simulink model "PMSM_SVC_HF"  (R2023a)
settings: Solver=ode1  StartTime=0.0  StopTime=7  FixedStep=Tsim  RelTol=1e-3  EnableMultiTasking=on
InitFcn:
  | %% Parameters of the motor
  | Pw_n = 1;                                                                   % The nominal power of the SM (kW)
  | Ull_n = 380;                                                                % The nominal line-line voltage (Vrms)
  | I_n = 2;                                                                    % The nominal current (A)
  | f_n = 50;                                                                   % The nominal frequency (Hz)
  | N_n = 1500;                                                                 % The nominal rotation speed of motor (rad.min^-1)
  | p = 2;                                                                      % Pole pairs
  | T_n = 5;                                                                    % The nominal torque of motor (N.m)
  | 
  | Rs = 0.91;                                                                  % The stator resistance (ohm)
  | Ld = 3.96e-3;                                                               % The d-axis inductance (H)
  | Lq = 7.96e-3;                                                               % The q-axis inductance (H)
  | Ls = (Ld+Lq)/2;                                                             % The stator inductance (H)
  | Flux = 0.446;                                                               % The peak value of flux-linkage established by magnets (Wb)
  | Jm = 0.074;                                                                 % Inertia of the rotor (kg.m^2)
  | Fr = 0.008;                                                                 % Friction factor (N.m.s)
  | 
  | %% Parameters of the frequency converter and power net
  | fpwm = 10e3;                                                                % The frequency of the pwm (Hz)
  | Udc = 600;                                                                  % The line-line voltage of power net (Vrms)
  | 
  | %% Simulation parameters
  | Tcur = 1/fpwm;                                                              % Sample time in current loop (s)
  | Tsim = Tcur/500;%Tcur;                                                                % Sample time for simulation (s)
  | 
  | %% Controller limiter
  | T_max = T_n*1.5;                                                            % Maximum torque (Nm)
  | i_max = I_n*2.0*sqrt(2);                                                    % Maximum current (A)
  | u_max = Udc/sqrt(3);                                                        % Maximum voltage (V)
  | 
  | %% High frequency injection parameters
  | f_HF = 1000;                                                                 % Injection signal frequency (Hz)
  | v_HF = 20;                                                                  % Injection signal amplitude (V)
  | bw_BPF = 100;                                                               % Bandpass filter bandwidth (Hz)
undefined symbols (not defined in the file or in its folder): DiscIntNeverNeededParam
libraries: simulink x2, dspfdesign x2, spsStairGeneratorLib x2, spsUniversalBridgeLib x1, spsSecondOrderFilterLib x1, powerlib_extras x1, spsPermanentMagnetSynchronousMachineLib x1, spsDCVoltageSourceLib x1, sps_lib x1
settings Model: DSRTSU_INTERNAL_RTI_VER=490  DSRTSU_INTERNAL_RTI_TYPE=rti1202  Creator=XIL1XI  LastModifiedBy=Guoguo
settings SolverCC: AlgebraicLoopSolver=TrustRegion  AutoInsertRateTranBlk=on
settings DataIOCC: LimitDataPoints=on  ReturnWorkspaceOutputs=off
settings OptimizationCC: BlockReduction=off  OptimizeBlockIOStorage=off  BufferReuse=off  GlobalBufferReuse=off  ExpressionFolding=off  LocalBlockOutputs=off  LifeSpan=inf  OptimizeDataStoreBuffers=off  BusAssignmentInplaceUpdate=off
settings DebuggingCC: UnconnectedInputMsg=warning  UnconnectedOutputMsg=warning  UnconnectedLineMsg=warning  AllowSymbolicDim=off  SFUnexpectedBacktrackingDiag=warning  SFNoUnconditionalDefaultTransitionDiag=warning  SFExecutionAtInitializationDiag=none  ArithmeticOperatorsInVariantConditions=warning
settings HardwareCC: ProdBitPerPointer=32  ProdBitPerSizeT=32  ProdBitPerPtrDiffT=32  ProdLargestAtomicInteger=Integer  ProdEndianess=BigEndian  ProdWordSize=32  ProdHWDeviceType=Custom Processor->Custom
settings ModelReferenceCC: EnableRefExpFcnMdlSchedulingChecks=on  PropagateSignalLabelsOutOfModel=off
settings SFSimCC: SimUseLocalCustomCode=off  CustomCodeUndefinedFunction=UseInterfaceOnly
settings RTWCC: Description=dSPACE DS1202 Hardware Platform  SystemTargetFile=rti1202.tlc  MakeCommand=make_rti  TemplateMakefile=rti1202.tmf  RTWUseLocalCustomCode=off
settings CodeAppCC: StateflowObjectComments=on
settings STFCustomTargetCC: TargetLangStandard=C89/C90 (ANSI)  ModelReferenceCompliant=off  ParMdlRefBuildCompliant=on  ConcurrentExecutionCompliant=off  MatFileLogging=on  GRTInterface=off  UseToolchainInfoCompliant=off  SystemTargetFile=rti1202.tlc
settings GRTTargetCC: TargetLangStandard=C89/C90 (ANSI)  ModelReferenceCompliant=off  CompOptLevelCompliant=off  ConcurrentExecutionCompliant=off  CombineOutputUpdateFcns=off  CPPClassGenCompliant=off  UseToolchainInfoCompliant=off
settings ConfigComp: CovMetricSettings=dw  CovSaveCumulativeToWorkspaceVar=on  CovSaveSingleToWorkspaceVar=on  CovExternalEMLEnable=off
settings SimscapeCC: SimscapeNormalizeSystem=off

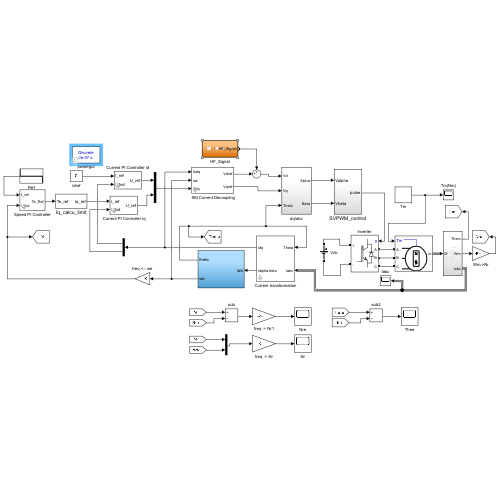
[thumbnail: Simulink's stored preview of the top-level diagram]
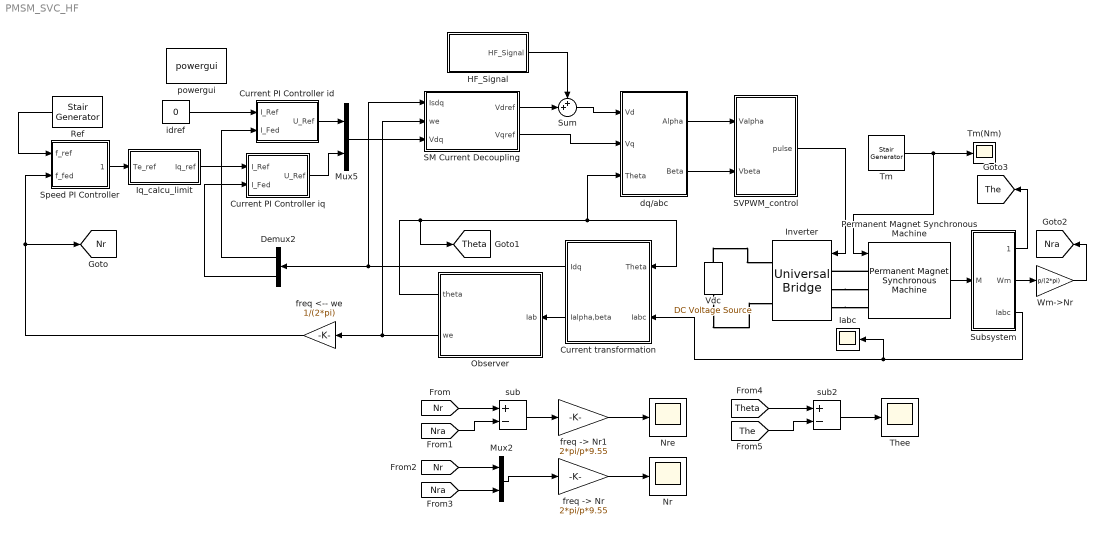
== system PMSM_SVC_HF ==
  " Current PI Controller iq" : Subsystem  mask(Current PI Controller){Rs=Rs, Ls=Ld, fpwm=fpwm, Par_Limits=[u_max -u_max], T=Tcur, kp_gain=1, ti_gain=1}
      mask prompts: Rs "Stator resistance Rs (ohm):"; Ls "Stator inductance Ls (H):"; fpwm "PWM frequency fpwm (Hz):"; Par_Limits "Output limits Par_Limits (V): [ Upper   Lower ]"; T "Sample time T (s):"
      mask help:
      | Kp, Ti can be calculated automatically:
      |
      |     kp = Ls/2*fpwm;
      |     ti = Ls/Rs;
      |     ki = kp/ti;
      |
      | Kp_Gain, Ki_Gain are used to adjust the calculated kp and ki. Controller limit is the integrator saturation limit and the output limit.
      mask Display:
      | port_label('input',1,'I_ref');
      | port_label('input',2,'I_fed');
      | port_label('output',1,'U_ref');
  " SM Current Decoupling" : Subsystem  mask(SM Feedforward Decoupling){Rs=Rs, Ls=Ls, Flux=Flux, Par_Limits=[u_max -u_max], T=Tcur}
      mask prompts: Rs "The stator resistance /ohm:"; Ls "The stator inductance /H:"; Flux "The flux linkage established by magnets /Wb"; Par_Limits "Output voltage limit (V): [ Upper  Lower ]"; T "Sample time T (s):"
      mask help:
      | This module is a current decoupling scheme:
      | -> Vd_Ref = Vd + (d-axis decoupling part)
      | -> Vq_Ref = Vq + (q-axis decoupling part)
      | The total output is limited according to parameter setting.
      mask init:
      | UpperLimit=Par_Limits(1);
      | LowerLimit=Par_Limits(2);
  Current PI Controller id : Subsystem  mask(Current PI Controller){Rs=Rs, Ls=Ld, fpwm=fpwm, Par_Limits=[u_max -u_max], T=Tcur, kp_gain=1, ti_gain=1}
      mask prompts: Rs "Stator resistance Rs (ohm):"; Ls "Stator inductance Ls (H):"; fpwm "PWM frequency fpwm (Hz):"; Par_Limits "Output limits Par_Limits (V): [ Upper   Lower ]"; T "Sample time T (s):"
      mask help:
      | Kp, Ti can be calculated automatically:
      |
      |     kp = Ls/2*fpwm;
      |     ti = Ls/Rs;
      |     ki = kp/ti;
      |
      | Kp_Gain, Ki_Gain are used to adjust the calculated kp and ki. Controller limit is the integrator saturation limit and the output limit.
      mask Display:
      | port_label('input',1,'I_ref');
      | port_label('input',2,'I_fed');
      | port_label('output',1,'U_ref');
  Current transformation : Subsystem  mask(Transformation abc to ab and dq){T=Tcur}
      mask prompts: T "Sample time T (s):"
  Demux2 : Demux  Outputs=2
  HF_Signal : Subsystem
  Iabc : Scope
  Inverter : spsUniversalBridgeLib/Universal Bridge  Arms=3  SnubberResistance=1e5  SnubberCapacitance=inf  Device=IGBT / Diodes  Ron=1e-3  Lon=0  ForwardVoltages=[0,0]  ForwardVoltage=0  GTOparameters=[ 10e-6 , 20e-6 ]  IGBTparameters=[0,0]  Measurements=None  Measurements_2=None  converterType=Rectifier
  Iq_calcu_limit : Subsystem
  Mux2 : Mux  Inputs=2
  Mux5 : Mux  Inputs=2
  Nr : Scope
  Nre : Scope
  Observer : Subsystem
  Permanent Magnet Synchronous Machine : spsPermanentMagnetSynchronousMachineLib/Permanent Magnet Synchronous Machine  NbPhases=3  FluxDistribution=Sinusoidal  RotorType=Salient-pole  MechanicalLoad=Torque Tm  PresetModel=No  ShowDetailedParameters=on  MeasurementBus=off  Resistance=Rs  Inductance=8.5e-3  dqInductances=[Ld,Lq]  La=Ls  MachineConstant=Flux linkage established by magnets (V.s)  Flux=Flux  VoltageCst=161.7909  TorqueCst=1.338  Flat=120  Mechanical=[Jm Fr p 0]  PolePairs=4  InitialConditions=[0,0, 0,0]  InitialConditions5ph=[0 0 0 0 0 0]  RefAngle=Aligned with phase A axis (original Park)  IterativeDiscreteModel=Trapezoidal non iterative  TsBlock=-1  TsPowergui=0
  Ref : spsStairGeneratorLib/Stair Generator  t="[0  0.5  4.5 ]"  e=[0 10 20]  Ts=Tcur
  SVPWM_control : Subsystem
  Speed PI Controller : Subsystem  mask(Speed PI Controller){kp=2.5, ti=2.5/10, Par_Limits=[T_max -T_max], T=Tcur}
      mask prompts: kp "proportional gain"; ti "integral time"; Par_Limits "Output limits: [ Upper   Lower ]"; T "Sample time T (s):"
      mask help:
      | Kp, Ti can be calculated automatically:
      |
      |     kp = Jm*(h+1)/(2*h*2*fpwm*kt)*kp_gain;
      |     ki = Jm*(h+1)/(2*h*2*fpwm*kt)/(2*1/fpwm)*ti_gain;
      |     ti = kp/ki;
      |
      |
      | Kp_Gain, Ki_Gain are used to adjust the calculated kp and ki. Controller limit is the integrator saturation limit and the output limit.
      mask init:
      | UpperLimit=Par_Limits(1);
      | LowerLimit=Par_Limits(2);
      | 
      | ki = kp/ti;
  Subsystem : Subsystem
  Sum : Sum  Inputs=++|
  Thee : Scope
  Tm : spsStairGeneratorLib/Stair Generator  t="[0  3.5 ]"  e=[0 3 ]  Ts=0
  Tm(Nm) : Scope
  Vdc : spsDCVoltageSourceLib/DC Voltage Source  Amplitude=Udc  Measurements=None
  Wm->Nr : Gain  Gain=p/(2*pi)
  dq/abc : Subsystem
  "freq -> Nr" : Gain  Gain=2*pi/p*9.55
  "freq -> Nr1" : Gain  Gain=2*pi/p*9.55
  freq <-- we : Gain  Gain=1/(2*pi)
  idref : Constant  Value=0
  powergui : sps_lib/powergui  Priority=1  SimulationMode=Discrete  SampleTime=Tsim  frequency=60  Iterations=50  frequencyindice=0  Pbase=100e6  ErrMax=1e-4  UnitsV=kV  UnitsW=MW  buscounter=0  FunctionMessages=off  echomessages=off  EnableUseOfTLC=off  CurrentSourceSwitches=off  DisableSnubberDevices=off  DisableRonSwitches=off  DisableVfSwitches=off  DisplayEquations=off  AutomaticDiscreteSolvers=off  SolverType=Tustin/Backward Euler (TBE)  Interpol=off  ExternalGateDelay=off  methode=off  Ts=10  x0status=blocks  SPID=off  SwTol=0  HookPort=off  NonlinearTolerance=1e-4  nMaxIteration=100  ContinueOnMaxIteration=off  RestoreLinks=warning  ResistiveCurrentMeasurement=off  Frange=[0:2:500]  Ylog=off  Xlog=on  ShowGrid=off  save=off  variable=ZData  structure=0  ZoomFFT=off  StartTime=0.0  cycles=1  DisplayStyle=1  fundamental=60  FreqAxis=off  MaxFrequency=1000  frequencyindicesteady=1  RmsSteady=1  display=off
  sub : Sum  Inputs=+-
  sub2 : Sum  Inputs=+-
  tag scope: Nr=global, Nra=global, The=global, Theta=global
  wires:
  Current PI Controller id/1(U_Ref) -> Mux5/1
  " Current PI Controller iq"/1(U_Ref) -> Mux5/2
  Observer/2(we) -> " SM Current Decoupling"/2(we), freq <-- we/1
  Mux2/1 -> "freq -> Nr"/1
  Iq_calcu_limit/1(Iq_ref) -> " Current PI Controller iq"/1(I_Ref)
  idref/1 -> Current PI Controller id/1(I_Ref)
  Speed PI Controller/1(Te_Ref) -> Iq_calcu_limit/1(Te_ref)
  Current transformation/1(Idq) -> Demux2/1, " SM Current Decoupling"/1(Isdq)
  Current transformation/2(Ialpha,beta) -> Observer/1(Iab)
  Tm/1 -> Permanent Magnet Synchronous Machine/1, Tm(Nm)/1
  sub/1 -> "freq -> Nr1"/1
  Ref/1 -> Speed PI Controller/1(f_ref)
  Permanent Magnet Synchronous Machine/1 -> Subsystem/1(M)
  Mux5/1 -> " SM Current Decoupling"/3(Vdq)
  Subsystem/3(Iabc) -> Iabc/1, Current transformation/2(Iabc)
  "freq -> Nr"/1 -> Nr/1
  "freq -> Nr1"/1 -> Nre/1
  Demux2/1 -> Current PI Controller id/2(I_Fed)
  Demux2/2 -> " Current PI Controller iq"/2(I_Fed)
  Subsystem/2(Wm) -> Wm->Nr/1
  Observer/1(theta) -> [Theta], Current transformation/1(Theta), dq/abc/3(Theta)
  freq <-- we/1 -> [Nr], Speed PI Controller/2(f_fed)
  [Nr] -> sub/1
  Wm->Nr/1 -> [Nra]
  [Nra] -> sub/2
  [Nr] -> Mux2/1
  [Nra] -> Mux2/2
  Subsystem/1(Them) -> [The]
  [Theta] -> sub2/1
  [The] -> sub2/2
  sub2/1 -> Thee/1
  dq/abc/1(Alpha) -> SVPWM_control/1(Valpha)
  dq/abc/2(Beta) -> SVPWM_control/2(Vbeta)
  SVPWM_control/1(pulse) -> Inverter/1
  HF_Signal/1(HF_Signal) -> Sum/1
  " SM Current Decoupling"/1(Vdref) -> Sum/2
  Sum/1 -> dq/abc/1(Vd)
  " SM Current Decoupling"/2(Vqref) -> dq/abc/2(Vq)
  connections:
  Inverter/LConn2 -- Permanent Magnet Synchronous Machine/LConn2
  Permanent Magnet Synchronous Machine/LConn1 -- Inverter/LConn1
  Inverter/LConn3 -- Permanent Magnet Synchronous Machine/LConn3
  Vdc/RConn1 -- Inverter/RConn1
  Vdc/LConn1 -- Inverter/RConn2

== system PMSM_SVC_HF/ Current PI Controller iq ==
  I_Ref : Inport
  I_Fed : Inport  Port=2
  Discrete-Time Integrator1 : DiscreteIntegrator  IntegratorMethod=Integration: Trapezoidal  SampleTime=T  LimitOutput=on  UpperSaturationLimit=Par_Limits(1)  LowerSaturationLimit=Par_Limits(2)  ICPrevOutput=DiscIntNeverNeededParam  ICPrevScaledInput=DiscIntNeverNeededParam
  Output limit : Saturate  UpperLimit=Par_Limits(1)  LowerLimit=Par_Limits(2)
  Sum : Sum  Inputs=|+-
  Sum1 : Sum  Inputs=|++
  ki : Gain  Gain=(Ls/2*fpwm)/(Ls/Rs)*kp_gain/ti_gain
  kp : Gain  Gain=(Ls/2*fpwm)*kp_gain
  U_Ref : Outport  VectorParamsAs1DForOutWhenUnconnected=off
  wires:
  kp/1 -> Sum1/1
  I_Ref/1 -> Sum/1
  I_Fed/1 -> Sum/2
  Sum/1 -> ki/1, kp/1
  Sum1/1 -> Output limit/1
  Output limit/1 -> U_Ref/1
  Discrete-Time Integrator1/1 -> Sum1/2
  ki/1 -> Discrete-Time Integrator1/1

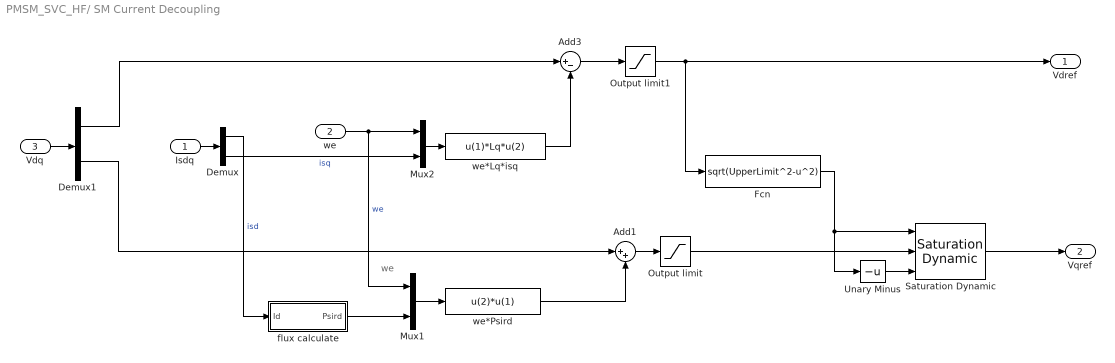
== system PMSM_SVC_HF/ SM Current Decoupling ==
  note: we
  Isdq : Inport
  we : Inport  Port=2
  Vdq : Inport  Port=3
  Add1 : Sum  Inputs=|++  SampleTime=T
  Add3 : Sum  Inputs=|+-  SampleTime=T
  Demux : Demux  Outputs=2
  Demux1 : Demux  Outputs=2
  Fcn : Fcn  Expr=sqrt(UpperLimit^2-u^2)
  Mux1 : Mux  Inputs=2
  Mux2 : Mux  Inputs=2
  Output limit : Saturate  UpperLimit=UpperLimit  LowerLimit=LowerLimit
  Output limit1 : Saturate  UpperLimit=UpperLimit  LowerLimit=LowerLimit
  Saturation Dynamic : simulink/Discontinuities/Saturation Dynamic  OutMin=[]  OutMax=[]  OutDataTypeStr=Inherit: Same as second input  OutDataType=fixdt(1, 16)  OutScaling=2^-10  DoSatur=off
  Unary Minus : UnaryMinus
  flux calculate : Subsystem
  we*Lq*isq : Fcn  Expr=u(1)*Lq*u(2)  SampleTime=T
  we*Psird : Fcn  Expr=u(2)*u(1)  SampleTime=T
  Vdref : Outport  VectorParamsAs1DForOutWhenUnconnected=off
  Vqref : Outport  Port=2  VectorParamsAs1DForOutWhenUnconnected=off
  wires:
  flux calculate/1(Psird) -> Mux1/2
  Demux1/2 -> Add1/1
  Add3/1 -> Output limit1/1
  we*Lq*isq/1 -> Add3/2
  Demux1/1 -> Add3/1
  Output limit1/1 -> Vdref/1, Fcn/1
  Vdq/1 -> Demux1/1
  Mux1/1 -> we*Psird/1
  we/1 -> Mux2/1, Mux1/1  "we"
  Mux2/1 -> we*Lq*isq/1
  Add1/1 -> Output limit/1
  Demux/2 -> Mux2/2  "isq"
  Demux/1 -> flux calculate/1(Id)  "isd"
  Fcn/1 -> Unary Minus/1, Saturation Dynamic/1
  Unary Minus/1 -> Saturation Dynamic/3
  Output limit/1 -> Saturation Dynamic/2
  we*Psird/1 -> Add1/2
  Isdq/1 -> Demux/1
  Saturation Dynamic/1 -> Vqref/1

== system PMSM_SVC_HF/Current PI Controller id ==
  I_Ref : Inport
  I_Fed : Inport  Port=2
  Discrete-Time Integrator1 : DiscreteIntegrator  IntegratorMethod=Integration: Trapezoidal  SampleTime=T  LimitOutput=on  UpperSaturationLimit=Par_Limits(1)  LowerSaturationLimit=Par_Limits(2)  ICPrevOutput=DiscIntNeverNeededParam  ICPrevScaledInput=DiscIntNeverNeededParam
  Output limit : Saturate  UpperLimit=Par_Limits(1)  LowerLimit=Par_Limits(2)
  Sum : Sum  Inputs=|+-
  Sum1 : Sum  Inputs=|++
  ki : Gain  Gain=(Ls/2*fpwm)/(Ls/Rs)*kp_gain/ti_gain
  kp : Gain  Gain=(Ls/2*fpwm)*kp_gain
  U_Ref : Outport  VectorParamsAs1DForOutWhenUnconnected=off
  wires:
  kp/1 -> Sum1/1
  I_Ref/1 -> Sum/1
  I_Fed/1 -> Sum/2
  Sum/1 -> ki/1, kp/1
  Sum1/1 -> Output limit/1
  Output limit/1 -> U_Ref/1
  Discrete-Time Integrator1/1 -> Sum1/2
  ki/1 -> Discrete-Time Integrator1/1

== system PMSM_SVC_HF/Current transformation ==
  Theta : Inport
  Iabc : Inport  Port=2
  2R Transform1 : Subsystem  mask(2S/2R Transform){}
      mask help:
      | -> D = Alpha *cos(Theta)+ Beta *sin(Theta)
      | -> Q = -Alpha *sin(Theta)+ Beta *cos(Theta)
      mask Display: fprintf('2S/2R', 17)
  3s/2s : Subsystem
  Mux6 : Mux  Inputs=2
  Rate Transition7 : RateTransition
  Zero-Order Hold6 : ZeroOrderHold  SampleTime=T
  Idq : Outport  VectorParamsAs1DForOutWhenUnconnected=off
  Ialpha,beta : Outport  Port=2  VectorParamsAs1DForOutWhenUnconnected=off
  wires:
  Iabc/1 -> Rate Transition7/1
  Zero-Order Hold6/1 -> 3s/2s/1(abc)
  3s/2s/1(alpha) -> Mux6/1
  3s/2s/2(beta) -> Mux6/2
  2R Transform1/1(DQ) -> Idq/1
  Mux6/1 -> Ialpha,beta/1, 2R Transform1/2(AB)
  Theta/1 -> 2R Transform1/1(Theta)
  Rate Transition7/1 -> Zero-Order Hold6/1

== system PMSM_SVC_HF/HF_Signal ==
  Cos Wave : Sin  Amplitude=v_HF  Frequency=2*pi*f_HF  Phase=pi/2  SampleTime=Tcur
  Rate Transition7 : RateTransition
  Zero-Order Hold6 : ZeroOrderHold  SampleTime=Tcur
  HF_Signal : Outport  VectorParamsAs1DForOutWhenUnconnected=off
  wires:
  Rate Transition7/1 -> Zero-Order Hold6/1
  Cos Wave/1 -> Rate Transition7/1
  Zero-Order Hold6/1 -> HF_Signal/1

== system PMSM_SVC_HF/Iq_calcu_limit ==
  Te_ref : Inport
  Fcn : Fcn  Expr=(2/3)*u/p/Flux
  Output limit1 : Saturate  UpperLimit=i_max  LowerLimit=-i_max
  Zero-Order Hold3 : ZeroOrderHold  SampleTime=Tcur
  Iq_ref : Outport  InitialOutput=0  VectorParamsAs1DForOutWhenUnconnected=off
  wires:
  Te_ref/1 -> Zero-Order Hold3/1
  Zero-Order Hold3/1 -> Fcn/1
  Fcn/1 -> Output limit1/1
  Output limit1/1 -> Iq_ref/1

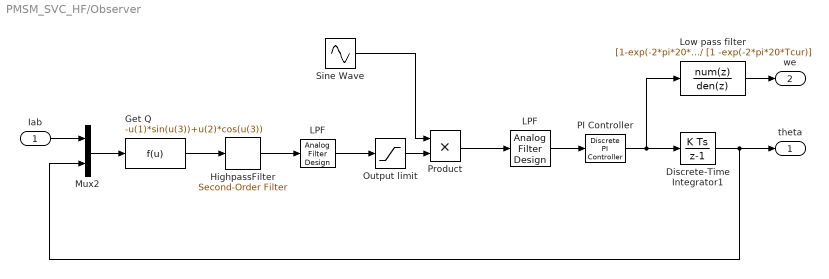
== system PMSM_SVC_HF/Observer ==
  Iab : Inport
  " LPF" : dspfdesign/Analog Filter Design  method=Butterworth  filttype=Lowpass  N=1  Wlo=2*pi*100  Whi=80  Rp=2  Rs=40
  Discrete-Time Integrator1 : DiscreteIntegrator  SampleTime=-1  ICPrevOutput=DiscIntNeverNeededParam  ICPrevScaledInput=DiscIntNeverNeededParam
  Get Q : Fcn  Expr=-u(1)*sin(u(3))+u(2)*cos(u(3))
  HighpassFilter : spsSecondOrderFilterLib/Second-Order Filter  FilterType=Highpass  Fo=f_HF - bw_BPF/2  Zeta=0.3  Ts=Tcur  Initialize=off  Vac_Init="[0,  0,  60]"  Vdc_Init=0  PlotResponse=off  FreqRange=[0, 10000, 1]
      settings: LibrarySourceBlock=|
      | sps_lib/Control/Filters/Second-Order
      | Filter
  LPF : dspfdesign/Analog Filter Design  method=Butterworth  filttype=Lowpass  N=2  Wlo=(f_HF + bw_BPF)*6.28  Whi=6360  Rp=2  Rs=40
  Low pass filter : DiscreteTransferFcn  Numerator=[1-exp(-2*pi*20*Tcur)]  Denominator=[1 -exp(-2*pi*20*Tcur)]  SampleTime=Tcur
  Mux2 : Mux  Inputs=2
  Output limit : Saturate
  PI Controller : powerlib_extras/Discrete  Control Blocks/Discrete PI Controller  Kp=5  Ki=50  Par_Limits=[100*2*pi -100*2*pi]  Init=0  Ts=Tcur
  Product : Product
  Sine Wave : Sin  Amplitude=v_HF  Frequency=2*pi*f_HF  SampleTime=Tcur
  theta : Outport  VectorParamsAs1DForOutWhenUnconnected=off
  we : Outport  Port=2  VectorParamsAs1DForOutWhenUnconnected=off
  wires:
  Iab/1 -> Mux2/1
  Get Q/1 -> HighpassFilter/1
  Product/1 -> " LPF"/1
  " LPF"/1 -> PI Controller/1
  PI Controller/1 -> Discrete-Time Integrator1/1, Low pass filter/1
  Output limit/1 -> Product/2
  HighpassFilter/1 -> LPF/1
  Discrete-Time Integrator1/1 -> theta/1, Mux2/2
  Mux2/1 -> Get Q/1
  Low pass filter/1 -> we/1
  Sine Wave/1 -> Product/1
  LPF/1 -> Output limit/1

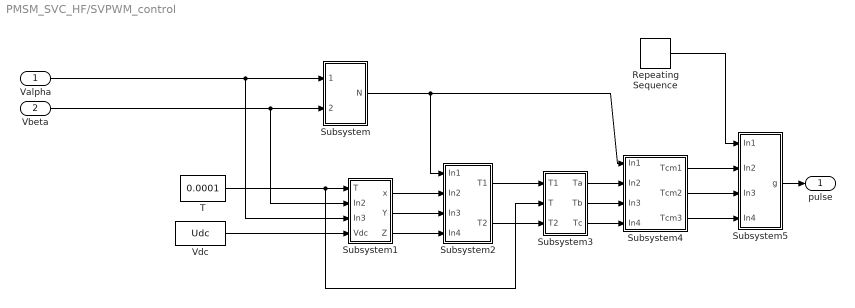
== system PMSM_SVC_HF/SVPWM_control ==
  Valpha : Inport
  Vbeta : Inport  Port=2
  Repeating Sequence : simulink/Sources/Repeating Sequence  rep_seq_t=[0 0.00005 0.0001]  rep_seq_y=[0 0.00005 0]
  Subsystem : Subsystem
  Subsystem1 : Subsystem
  Subsystem2 : Subsystem
  Subsystem3 : Subsystem
  Subsystem4 : Subsystem
  Subsystem5 : Subsystem
  T : Constant  Value=0.0001
  Vdc : Constant  Value=Udc
  pulse : Outport  VectorParamsAs1DForOutWhenUnconnected=off
  wires:
  Subsystem5/1(g) -> pulse/1
  Repeating Sequence/1 -> Subsystem5/1(In1)
  Subsystem4/3(Tcm3) -> Subsystem5/4(In4)
  Subsystem4/2(Tcm2) -> Subsystem5/3(In3)
  Subsystem4/1(Tcm1) -> Subsystem5/2(In2)
  Subsystem3/3(Tc) -> Subsystem4/4(In4)
  Subsystem3/2(Tb) -> Subsystem4/3(In3)
  Subsystem3/1(Ta) -> Subsystem4/2(In2)
  Subsystem2/2(T2) -> Subsystem3/3(T2)
  Subsystem2/1(T1) -> Subsystem3/1(T1)
  Subsystem1/3(Z) -> Subsystem2/4(In4)
  Subsystem1/2(Y) -> Subsystem2/3(In3)
  Subsystem1/1(x) -> Subsystem2/2(In2)
  Subsystem/1(N) -> Subsystem4/1(In1), Subsystem2/1(In1)
  Vdc/1 -> Subsystem1/4(Vdc)
  T/1 -> Subsystem3/2(T), Subsystem1/1(T)
  Vbeta/1 -> Subsystem1/2(In2), Subsystem/2(Vbeta)
  Valpha/1 -> Subsystem1/3(In3), Subsystem/1(Valpha)

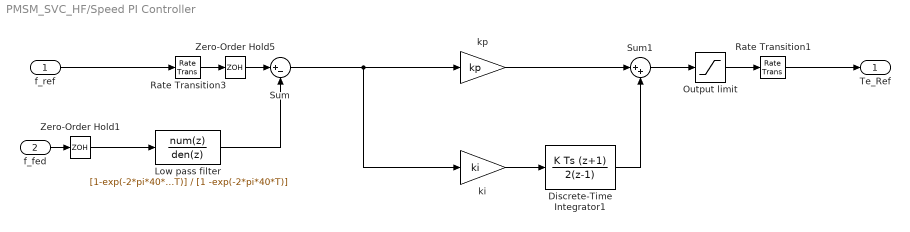
== system PMSM_SVC_HF/Speed PI Controller ==
  f_ref : Inport
  f_fed : Inport  Port=2
  Discrete-Time Integrator1 : DiscreteIntegrator  IntegratorMethod=Integration: Trapezoidal  SampleTime=T  LimitOutput=on  UpperSaturationLimit=UpperLimit  LowerSaturationLimit=LowerLimit  ICPrevOutput=DiscIntNeverNeededParam  ICPrevScaledInput=DiscIntNeverNeededParam
  Low pass filter : DiscreteTransferFcn  Numerator=[1-exp(-2*pi*40*T)]  Denominator=[1 -exp(-2*pi*40*T)]  SampleTime=T
  Output limit : Saturate  UpperLimit=UpperLimit  LowerLimit=LowerLimit
  Rate Transition1 : RateTransition
  Rate Transition3 : RateTransition
  Sum : Sum  Inputs=|+-
  Sum1 : Sum  Inputs=|++
  Zero-Order Hold1 : ZeroOrderHold  SampleTime=T
  Zero-Order Hold5 : ZeroOrderHold  SampleTime=T
  ki : Gain  Gain=ki
  kp : Gain  Gain=kp
  Te_Ref : Outport  VectorParamsAs1DForOutWhenUnconnected=off
  wires:
  ki/1 -> Discrete-Time Integrator1/1
  Discrete-Time Integrator1/1 -> Sum1/2
  Sum1/1 -> Output limit/1
  Sum/1 -> kp/1, ki/1
  kp/1 -> Sum1/1
  f_ref/1 -> Rate Transition3/1
  Rate Transition3/1 -> Zero-Order Hold5/1
  Zero-Order Hold5/1 -> Sum/1
  f_fed/1 -> Zero-Order Hold1/1
  Zero-Order Hold1/1 -> Low pass filter/1
  Output limit/1 -> Rate Transition1/1
  Rate Transition1/1 -> Te_Ref/1
  Low pass filter/1 -> Sum/2

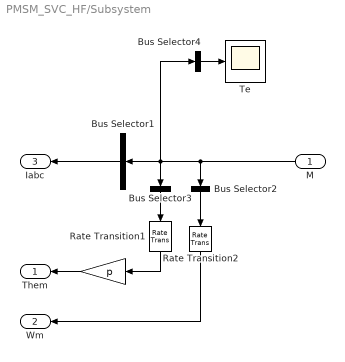
== system PMSM_SVC_HF/Subsystem ==
  M : Inport
  " " : Gain  Gain=p  SaturateOnIntegerOverflow=on  OutDataTypeStr=Inherit: Same as input  ParamDataTypeStr=Inherit: Same as input
  Bus Selector1 : BusSelector  OutputSignals=Stator current is_a (A),Stator current is_b (A),Stator current is_c (A)  OutputAsBus=on
  Bus Selector2 : BusSelector  OutputSignals=Rotor speed wm (rad/s)  OutputAsBus=on
  Bus Selector3 : BusSelector  OutputSignals=Rotor angle thetam (rad)  OutputAsBus=on
  Bus Selector4 : BusSelector  OutputSignals=Electromagnetic torque Te (N*m)  OutputAsBus=on
  Rate Transition1 : RateTransition  OutPortSampleTime=Tcur
  Rate Transition2 : RateTransition  OutPortSampleTime=Tcur
  Te : Scope
  Them : Outport  VectorParamsAs1DForOutWhenUnconnected=off
  Wm : Outport  Port=2  VectorParamsAs1DForOutWhenUnconnected=off
  Iabc : Outport  Port=3  VectorParamsAs1DForOutWhenUnconnected=off
  wires:
  M/1 -> Bus Selector4/1, Bus Selector3/1, Bus Selector1/1, Bus Selector2/1
  Bus Selector3/1 -> Rate Transition1/1
  Bus Selector1/1 -> Iabc/1
  Bus Selector2/1 -> Rate Transition2/1
  Rate Transition2/1 -> Wm/1
  Rate Transition1/1 -> " "/1
  " "/1 -> Them/1
  Bus Selector4/1 -> Te/1

== system PMSM_SVC_HF/dq//abc ==
  Vd : Inport
  Vq : Inport  Port=2
  Theta : Inport  Port=3
  Fcn : Fcn  Expr=u(1)*u(4)-u(2)*u(3)
  Fcn1 : Fcn  Expr=u(1)*u(3)+u(2)*u(4)
  Mux : Mux
  Trigonometric Function : Trigonometry
  Trigonometric Function1 : Trigonometry  Operator=cos
  Alpha : Outport  VectorParamsAs1DForOutWhenUnconnected=off
  Beta : Outport  Port=2  VectorParamsAs1DForOutWhenUnconnected=off
  wires:
  Theta/1 -> Trigonometric Function1/1, Trigonometric Function/1
  Trigonometric Function1/1 -> Mux/4
  Trigonometric Function/1 -> Mux/3
  Vq/1 -> Mux/2
  Vd/1 -> Mux/1
  Mux/1 -> Fcn1/1, Fcn/1
  Fcn/1 -> Alpha/1
  Fcn1/1 -> Beta/1

== system PMSM_SVC_HF/ SM Current Decoupling/flux calculate ==
  Id : Inport
  Add2 : Sum  SampleTime=T
  Flux : Constant  Value=Flux
  Ld*id : Fcn  Expr=Ld*u(1)  SampleTime=T
  Scope5 : Scope
  Psird : Outport  VectorParamsAs1DForOutWhenUnconnected=off
  wires:
  Flux/1 -> Add2/2
  Add2/1 -> Psird/1, Scope5/1
  Ld*id/1 -> Add2/1
  Id/1 -> Ld*id/1

== system PMSM_SVC_HF/Current transformation/2R Transform1 ==
  Theta : Inport
  AB : Inport  Port=2
  Get D : Fcn  Expr=u(1)*u(4)+u(2)*u(3)
  Get Q : Fcn  Expr=-u(1)*u(3)+u(2)*u(4)
  Mux : Mux  Inputs=2
  Mux2 : Mux  Inputs=2
  Sincos1 : Subsystem  mask(2S/2R Transform){}
      mask help:
      | -> D = Alpha *cos(Theta)+ Beta *sin(Theta)
      | -> Q = -Alpha *sin(Theta)+ Beta *cos(Theta)
  DQ : Outport  VectorParamsAs1DForOutWhenUnconnected=off
  wires:
  Mux/1 -> DQ/1
  Get Q/1 -> Mux/2
  Get D/1 -> Mux/1
  Mux2/1 -> Get D/1, Get Q/1
  AB/1 -> Mux2/1
  Theta/1 -> Sincos1/1(Theta)
  Sincos1/1(sincos theta) -> Mux2/2

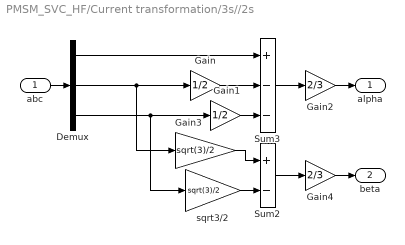
== system PMSM_SVC_HF/Current transformation/3s//2s ==
  abc : Inport
  Demux : Demux  Outputs=3
      settings: DisplayOption=none
  Gain : Gain  Gain=1/2  SaturateOnIntegerOverflow=on  OutDataTypeStr=Inherit: Same as input  ParamDataTypeStr=Inherit: Same as input
  Gain1 : Gain  Gain=1/2  SaturateOnIntegerOverflow=on  OutDataTypeStr=Inherit: Same as input  ParamDataTypeStr=Inherit: Same as input
  Gain2 : Gain  Gain=2/3  SaturateOnIntegerOverflow=on  OutDataTypeStr=Inherit: Same as input  ParamDataTypeStr=Inherit: Same as input
  Gain3 : Gain  Gain=sqrt(3)/2  SaturateOnIntegerOverflow=on  OutDataTypeStr=Inherit: Same as input  ParamDataTypeStr=Inherit: Same as input
  Gain4 : Gain  Gain=2/3  SaturateOnIntegerOverflow=on  OutDataTypeStr=Inherit: Same as input  ParamDataTypeStr=Inherit: Same as input
  Sum2 : Sum  Inputs=+-  InputSameDT=on  SaturateOnIntegerOverflow=on  OutDataTypeStr=Inherit: Same as first input
  Sum3 : Sum  Inputs=+--  InputSameDT=on  SaturateOnIntegerOverflow=on  OutDataTypeStr=Inherit: Same as first input
  sqrt3/2 : Gain  Gain=sqrt(3)/2  SaturateOnIntegerOverflow=on  OutDataTypeStr=Inherit: Same as input  ParamDataTypeStr=Inherit: Same as input
  alpha : Outport  VectorParamsAs1DForOutWhenUnconnected=off
  beta : Outport  Port=2  VectorParamsAs1DForOutWhenUnconnected=off
  wires:
  Sum2/1 -> Gain4/1
  Gain2/1 -> alpha/1
  abc/1 -> Demux/1
  Demux/1 -> Sum3/1
  Demux/2 -> Gain/1, Gain3/1
  Gain1/1 -> Sum3/3
  Gain/1 -> Sum3/2
  Demux/3 -> Gain1/1, sqrt3/2/1
  Gain3/1 -> Sum2/1
  sqrt3/2/1 -> Sum2/2
  Gain4/1 -> beta/1
  Sum3/1 -> Gain2/1

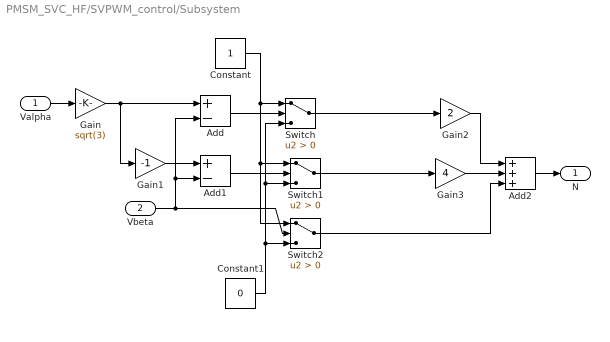
== system PMSM_SVC_HF/SVPWM_control/Subsystem ==
  Valpha : Inport
  Vbeta : Inport  Port=2
  Add : Sum  Inputs=+-
  Add1 : Sum  Inputs=+-
  Add2 : Sum  Inputs=+++
  Constant : Constant
  Constant1 : Constant  Value=0
  Gain : Gain  Gain=sqrt(3)
  Gain1 : Gain  Gain=-1
  Gain2 : Gain  Gain=2
  Gain3 : Gain  Gain=4
  Switch : Switch  Criteria=u2 > Threshold  SaturateOnIntegerOverflow=off  InputSameDT=off
  Switch1 : Switch  Criteria=u2 > Threshold  SaturateOnIntegerOverflow=off  InputSameDT=off
  Switch2 : Switch  Criteria=u2 > Threshold  SaturateOnIntegerOverflow=off  InputSameDT=off
  N : Outport  VectorParamsAs1DForOutWhenUnconnected=off
  wires:
  Add2/1 -> N/1
  Valpha/1 -> Gain/1
  Gain3/1 -> Add2/2
  Gain2/1 -> Add2/1
  Add1/1 -> Switch1/2
  Gain1/1 -> Add1/1
  Switch1/1 -> Gain3/1
  Switch2/1 -> Add2/3
  Switch/1 -> Gain2/1
  Add/1 -> Switch/2
  Gain/1 -> Gain1/1, Add/1
  Constant1/1 -> Switch/3, Switch1/3, Switch2/3
  Constant/1 -> Switch1/1, Switch2/1, Switch/1
  Vbeta/1 -> Add1/2, Add/2, Switch2/2

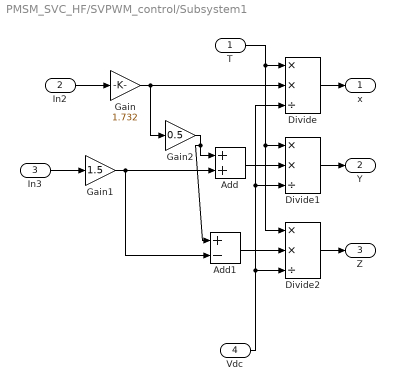
== system PMSM_SVC_HF/SVPWM_control/Subsystem1 ==
  T : Inport
  In2 : Inport  Port=2
  In3 : Inport  Port=3
  Vdc : Inport  Port=4
  Add : Sum
  Add1 : Sum  Inputs=+-
  Divide : Product  Inputs=**/
  Divide1 : Product  Inputs=**/
  Divide2 : Product  Inputs=**/
  Gain : Gain  Gain=1.732
  Gain1 : Gain  Gain=1.5
  Gain2 : Gain  Gain=0.5
  x : Outport  VectorParamsAs1DForOutWhenUnconnected=off
  Y : Outport  Port=2  VectorParamsAs1DForOutWhenUnconnected=off
  Z : Outport  Port=3  VectorParamsAs1DForOutWhenUnconnected=off
  wires:
  Divide2/1 -> Z/1
  Divide1/1 -> Y/1
  Divide/1 -> x/1
  In3/1 -> Gain1/1
  In2/1 -> Gain/1
  Add1/1 -> Divide2/2
  Add/1 -> Divide1/2
  Gain1/1 -> Add1/2, Add/2
  Gain2/1 -> Add1/1, Add/1
  Gain/1 -> Gain2/1, Divide/2
  Vdc/1 -> Divide/3, Divide1/3, Divide2/3
  T/1 -> Divide2/1, Divide1/1, Divide/1

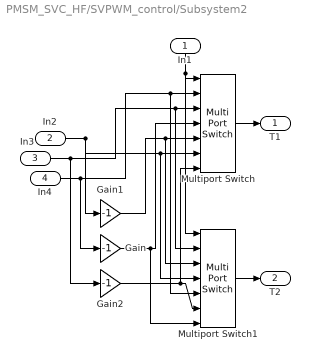
== system PMSM_SVC_HF/SVPWM_control/Subsystem2 ==
  In1 : Inport
  In2 : Inport  Port=2
  In3 : Inport  Port=3
  In4 : Inport  Port=4
  Gain : Gain  Gain=-1
  Gain1 : Gain  Gain=-1
  Gain2 : Gain  Gain=-1
  Multiport Switch : MultiPortSwitch  Inputs=6  SaturateOnIntegerOverflow=off  InputSameDT=off
  Multiport Switch1 : MultiPortSwitch  Inputs=6  SaturateOnIntegerOverflow=off  InputSameDT=off
  T1 : Outport  VectorParamsAs1DForOutWhenUnconnected=off
  T2 : Outport  Port=2  VectorParamsAs1DForOutWhenUnconnected=off
  wires:
  Multiport Switch1/1 -> T2/1
  Multiport Switch/1 -> T1/1
  Gain2/1 -> Multiport Switch/7, Multiport Switch1/6
  Gain1/1 -> Multiport Switch1/3, Multiport Switch/5
  In2/1 -> Gain1/1, Multiport Switch/6, Multiport Switch1/4
  Gain/1 -> Multiport Switch1/7, Multiport Switch/4
  In3/1 -> Gain2/1, Multiport Switch1/2, Multiport Switch/3
  In4/1 -> Gain/1, Multiport Switch/2, Multiport Switch1/5
  In1/1 -> Multiport Switch/1, Multiport Switch1/1

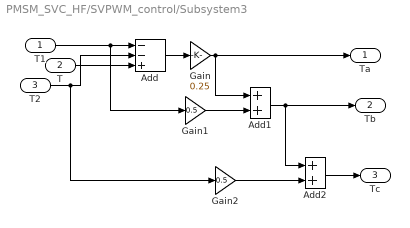
== system PMSM_SVC_HF/SVPWM_control/Subsystem3 ==
  T1 : Inport
  T : Inport  Port=2
  T2 : Inport  Port=3
  Add : Sum  Inputs=--+
  Add1 : Sum
  Add2 : Sum
  Gain : Gain  Gain=0.25
  Gain1 : Gain  Gain=0.5
  Gain2 : Gain  Gain=0.5
  Ta : Outport  VectorParamsAs1DForOutWhenUnconnected=off
  Tb : Outport  Port=2  VectorParamsAs1DForOutWhenUnconnected=off
  Tc : Outport  Port=3  VectorParamsAs1DForOutWhenUnconnected=off
  wires:
  T/1 -> Add/3
  Add2/1 -> Tc/1
  Gain2/1 -> Add2/2
  Add1/1 -> Add2/1, Tb/1
  Gain1/1 -> Add1/2
  Gain/1 -> Add1/1, Ta/1
  Add/1 -> Gain/1
  T2/1 -> Add/2, Gain2/1
  T1/1 -> Add/1, Gain1/1

== system PMSM_SVC_HF/SVPWM_control/Subsystem4 ==
  In1 : Inport
  In2 : Inport  Port=2
  In3 : Inport  Port=3
  In4 : Inport  Port=4
  Multiport Switch : MultiPortSwitch  Inputs=6  SaturateOnIntegerOverflow=off  InputSameDT=off
  Multiport Switch1 : MultiPortSwitch  Inputs=6  SaturateOnIntegerOverflow=off  InputSameDT=off
  Multiport Switch2 : MultiPortSwitch  Inputs=6  SaturateOnIntegerOverflow=off  InputSameDT=off
  Tcm1 : Outport  VectorParamsAs1DForOutWhenUnconnected=off
  Tcm2 : Outport  Port=2  VectorParamsAs1DForOutWhenUnconnected=off
  Tcm3 : Outport  Port=3  VectorParamsAs1DForOutWhenUnconnected=off
  wires:
  Multiport Switch2/1 -> Tcm3/1
  Multiport Switch1/1 -> Tcm2/1
  Multiport Switch/1 -> Tcm1/1
  In1/1 -> Multiport Switch2/1, Multiport Switch1/1, Multiport Switch/1
  In4/1 -> Multiport Switch1/3, Multiport Switch1/7, Multiport Switch2/2, Multiport Switch2/4, Multiport Switch/5, Multiport Switch/6
  In2/1 -> Multiport Switch/4, Multiport Switch/3, Multiport Switch1/2, Multiport Switch1/6, Multiport Switch2/5, Multiport Switch2/7
  In3/1 -> Multiport Switch/2, Multiport Switch/7, Multiport Switch1/4, Multiport Switch1/5, Multiport Switch2/3, Multiport Switch2/6

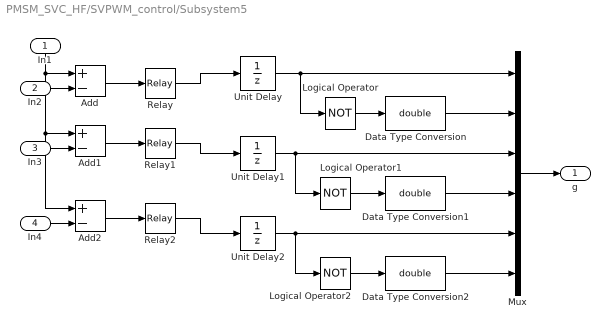
== system PMSM_SVC_HF/SVPWM_control/Subsystem5 ==
  In1 : Inport
  In2 : Inport  Port=2
  In3 : Inport  Port=3
  In4 : Inport  Port=4
  Add : Sum  Inputs=+-
  Add1 : Sum  Inputs=+-
  Add2 : Sum  Inputs=+-
  Data Type Conversion : DataTypeConversion  OutDataTypeStr=double  SaturateOnIntegerOverflow=off  RndMeth=Floor
  Data Type Conversion1 : DataTypeConversion  OutDataTypeStr=double  SaturateOnIntegerOverflow=off  RndMeth=Floor
  Data Type Conversion2 : DataTypeConversion  OutDataTypeStr=double  SaturateOnIntegerOverflow=off  RndMeth=Floor
  Logical Operator : Logic  Operator=NOT  AllPortsSameDT=off  OutDataTypeStr=boolean
  Logical Operator1 : Logic  Operator=NOT  AllPortsSameDT=off  OutDataTypeStr=boolean
  Logical Operator2 : Logic  Operator=NOT  AllPortsSameDT=off  OutDataTypeStr=boolean
  Mux : Mux  Inputs=6
  Relay : Relay  OffSwitchValue=-eps
  Relay1 : Relay  OffSwitchValue=-eps
  Relay2 : Relay  OffSwitchValue=-eps
  Unit Delay : UnitDelay  SampleTime=-1  HasFrameUpgradeWarning=on
  Unit Delay1 : UnitDelay  SampleTime=-1  HasFrameUpgradeWarning=on
  Unit Delay2 : UnitDelay  SampleTime=-1  HasFrameUpgradeWarning=on
  g : Outport  VectorParamsAs1DForOutWhenUnconnected=off
  wires:
  In4/1 -> Add2/2
  In3/1 -> Add1/2
  In2/1 -> Add/2
  Relay2/1 -> Unit Delay2/1
  Relay1/1 -> Unit Delay1/1
  Relay/1 -> Unit Delay/1
  Unit Delay2/1 -> Mux/5, Logical Operator2/1
  Unit Delay1/1 -> Mux/3, Logical Operator1/1
  Unit Delay/1 -> Logical Operator/1, Mux/1
  Mux/1 -> g/1
  Data Type Conversion/1 -> Mux/2
  Data Type Conversion1/1 -> Mux/4
  Data Type Conversion2/1 -> Mux/6
  Logical Operator2/1 -> Data Type Conversion2/1
  Logical Operator1/1 -> Data Type Conversion1/1
  Logical Operator/1 -> Data Type Conversion/1
  Add1/1 -> Relay1/1
  Add2/1 -> Relay2/1
  Add/1 -> Relay/1
  In1/1 -> Add/1, Add2/1, Add1/1

== system PMSM_SVC_HF/Current transformation/2R Transform1/Sincos1 ==
  Theta : Inport
  Mux2 : Mux  Inputs=2
  Trigonometric Function : Trigonometry
  Trigonometric Function1 : Trigonometry  Operator=cos
  sincos theta : Outport  VectorParamsAs1DForOutWhenUnconnected=off
  wires:
  Mux2/1 -> sincos theta/1
  Theta/1 -> Trigonometric Function/1, Trigonometric Function1/1
  Trigonometric Function/1 -> Mux2/1
  Trigonometric Function1/1 -> Mux2/2
